simulink model "fixpt_sl_dtc"  (Simulink 7.9)
settings: Solver=FixedStepDiscrete  StartTime=0.0  StopTime=0  FixedStep=1  RelTol=1e-3
settings Model: Creator=y_yama  LastModifiedBy=amatsumo
settings DataIOCC: SaveOutput=off  SignalLogging=off  SaveTime=off
settings OptimizationCC: InlineParams=on  InlineInvariantSignals=on  ZeroExternalMemoryAtStartup=off  ZeroInternalMemoryAtStartup=off  InitFltsAndDblsToZero=on  NoFixptDivByZeroProtection=on  EfficientFloat2IntCast=on  OptimizeModelRefInitCode=on  LifeSpan=1
settings DebuggingCC: InheritedTsInSrcMsg=none  FcnCallInpInsideContextMsg=Use local settings  StrictBusMsg=Warning
settings HardwareCC: ProdIntDivRoundTo=Zero  ProdEndianess=LittleEndian  ProdHWDeviceType=Generic->32-bit Embedded Processor
settings RTWCC: SystemTargetFile=ert.tlc  GenCodeOnly=on  TemplateMakefile=ert_default_tmf  Description=Real-Time Workshop Embedded Coder (no auto configuration)  GenerateReport=on  ProcessScript=ert_make_rtw_hook  IncludeHyperlinkInReport=on  LaunchReport=on
settings CodeAppCC: GenerateComments=off  IgnoreCustomStorageClasses=off  CustomSymbolStrGlobalVar=$N$M  SimulinkBlockComments=off
settings ERTTargetCC: CodeReplacementLibrary=ANSI_C  MultiwordLength=2048  GenerateSampleERTMain=on  IncludeMdlTerminateFcn=off  SuppressErrorStatus=on  SupportAbsoluteTime=off  SupportNonFinite=off  SupportComplex=off  PurelyIntegerCode=on  InlinedParameterPlacement=NonHierarchical  ERTCustomFileTemplate=example_file_process.tlc  ConvertIfToSwitch=off  SuppressUnreachableDefaultCases=off

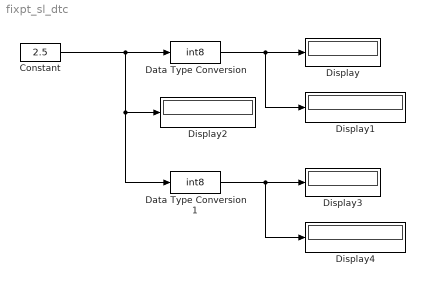
== system fixpt_sl_dtc ==
  Constant : Constant  Value=2.5  OutDataTypeStr=fixdt(1,8,1)  SampleTime=-1
      settings: AttributesFormatString=DataType = %<OutDataTypeStr>
  Data Type Conversion : DataTypeConversion  OutDataTypeStr=int8  RndMeth=Nearest
      settings: AttributesFormatString=DataType = %<OutDataTypeStr>
  Data Type Conversion1 : DataTypeConversion  OutDataTypeStr=int8  ConvertRealWorld=Stored Integer (SI)  RndMeth=Nearest
      settings: AttributesFormatString=DataType = %<OutDataTypeStr>
  Display{,1..4} (5 alike) : Display
      Display settings: AttributesFormatString=Format = %<Format>
      Display1 settings: AttributesFormatString=Format = %<Format>  Format=binary (Stored Integer)
      Display2 settings: AttributesFormatString=Format = %<Format>  Format=binary (Stored Integer)
      Display3 settings: AttributesFormatString=Format = %<Format>
      Display4 settings: AttributesFormatString=Format = %<Format>  Format=binary (Stored Integer)
  wires:
  Constant/1 -> Data Type Conversion/1, Display2/1, Data Type Conversion1/1
  Data Type Conversion/1 -> Display/1, Display1/1
  Data Type Conversion1/1 -> Display3/1, Display4/1
